simulink model "scattering_pos_pos_denis_2022a"  (R2022a)
settings: Solver=VariableStepAuto  StartTime=0.0  StopTime=10.0  RelTol=1e-3
values from neighbouring files (symbols this model uses):
  A = 2    [scattering_params.m]    (also in scattering_params_force_pos.m = 3; scattering_params_pos_pos.m = 3)
  b = 1    [scattering_params.m]    (also in scattering_params_force_pos.m = 40; scattering_params_pos_pos.m = 100)
  Be = 100    [scattering_params.m]    (also in scattering_params_force_pos.m; scattering_params_pos_pos.m)
  Bh = 1.5    [scattering_params.m]    (also in scattering_params_force_pos.m = 1; scattering_params_pos_pos.m = 1)
  Dh = 0.1    [scattering_params.m]    (also in scattering_params_force_pos.m = 16; scattering_params_pos_pos.m = 16)
  discrete_delay = 100    [scattering_params_force_pos.m]    (also in scattering_params_pos_pos.m)
  Dm = 0    [scattering_params.m]    (also in scattering_params_force_pos.m; scattering_params_pos_pos.m)
  Ds = 0    [scattering_params.m]    (also in scattering_params_force_pos.m; scattering_params_pos_pos.m)
  Fc = 1    [scattering_params.m]    (also in scattering_params_force_pos.m = 0.25; scattering_params_pos_pos.m = 0.25)
  Flp = 5    [scattering_params.m]    (also in scattering_params_force_pos.m = 0.5; scattering_params_pos_pos.m = 0.5)
  Jh = 1    [scattering_params.m]    (also in scattering_params_force_pos.m; scattering_params_pos_pos.m)
  Ke = 200    [scattering_params.m]    (also in scattering_params_force_pos.m; scattering_params_pos_pos.m)
  Mm = 0.5    [scattering_params.m]    (also in scattering_params_force_pos.m; scattering_params_pos_pos.m)
  Ms = 2    [scattering_params.m]    (also in scattering_params_force_pos.m; scattering_params_pos_pos.m)
  Ph = 10    [scattering_params.m]    (also in scattering_params_force_pos.m; scattering_params_pos_pos.m)
  scattering_filter_freq = 10    [scattering_params.m]    (also in scattering_params_force_pos.m; scattering_params_pos_pos.m)
  Ts = 0.001    [scattering_params_force_pos.m]    (also in scattering_params_pos_pos.m)
  xe = 5    [scattering_params.m]    (also in scattering_params_force_pos.m = 2; scattering_params_pos_pos.m = 2)
settings Model: Creator=Manu  LastModifiedBy=Manu
settings ModelReferenceCC: EnableRefExpFcnMdlSchedulingChecks=off
settings RTWCC: Description=Generic Real-Time Target

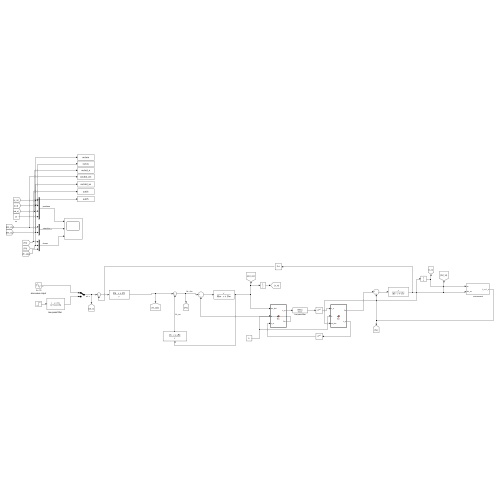
[thumbnail: Simulink's stored preview of the top-level diagram]
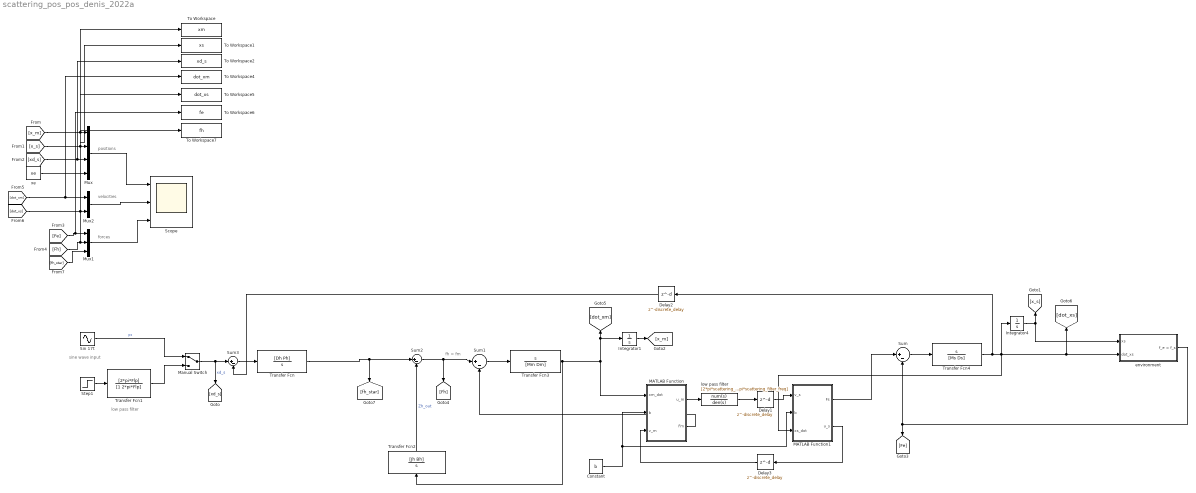
== system scattering_pos_pos_denis_2022a ==
  note: fh = fm
  note: sine wave input
  note: low pass filter
  note: positions
  note: forces
  note: velocities
  Constant : Constant  Value=b
  Delay1 : Delay  DelayLength=discrete_delay  SampleTime=Ts
  Delay2 : Delay  DelayLength=discrete_delay  SampleTime=Ts
  Delay3 : Delay  DelayLength=discrete_delay  SampleTime=Ts
  Integrator1 : Integrator
  Integrator4 : Integrator
  MATLAB Function : MATLAB Function  TreatAsAtomicUnit=on
  MATLAB Function1 : MATLAB Function  TreatAsAtomicUnit=on
  Manual Switch : ManualSwitch
  Mux : Mux
  Mux1 : Mux  Inputs=3
  Mux2 : Mux  Inputs=2
  Scope : Scope  NumInputPorts=3
  Sin 17t : Sin  Amplitude=A  Frequency=2*pi*Fc  SampleTime=0
  Step1 : Step  Time=0.5  After=A  SampleTime=0
  Sum{,1..3} (4 alike) : Sum  Inputs=|+-
  To Workspace : ToWorkspace  VariableName=xm  SaveFormat=Timeseries  SampleTime=-1
  To Workspace1 : ToWorkspace  VariableName=xs  SaveFormat=Timeseries  SampleTime=-1
  To Workspace2 : ToWorkspace  VariableName=xd_s  SaveFormat=Timeseries  SampleTime=-1
  To Workspace4 : ToWorkspace  VariableName=dot_xm  SaveFormat=Timeseries  SampleTime=-1
  To Workspace5 : ToWorkspace  VariableName=dot_xs  SaveFormat=Timeseries  SampleTime=-1
  To Workspace6 : ToWorkspace  VariableName=fe  SaveFormat=Timeseries  SampleTime=-1
  To Workspace7 : ToWorkspace  VariableName=fh  SaveFormat=Timeseries  SampleTime=-1
  Transfer Fcn : TransferFcn  Numerator=[Dh Ph]  Denominator=[1 0]
  Transfer Fcn1 : TransferFcn  Numerator=[2*pi*Flp]  Denominator=[1 2*pi*Flp]
  Transfer Fcn2 : TransferFcn  Numerator=[Jh Bh]  Denominator=[1 0]
  Transfer Fcn3 : TransferFcn  Numerator=[1 0]  Denominator=[Mm Dm]
  Transfer Fcn4 : TransferFcn  Numerator=[1 0]  Denominator=[Ms Ds]
  environment : Subsystem
  low pass filter : TransferFcn  Numerator=[2*pi*scattering_filter_freq]  Denominator=[1 2*pi*scattering_filter_freq]
  xe : Constant  Value=xe
  wires:
  Manual Switch/1 -> Sum3/1, [xd_s]  "xd_s"
  Transfer Fcn2/1 -> Sum2/2  "Zh_out"
  Sin 17t/1 -> Manual Switch/1  "F*"
  Transfer Fcn1/1 -> Manual Switch/2
  Step1/1 -> Transfer Fcn1/1
  Sum2/1 -> [Fh], Sum1/1
  Sum1/1 -> Transfer Fcn3/1
  Sum/1 -> Transfer Fcn4/1
  Transfer Fcn4/1 -> MATLAB Function1/3(xs_dot), [dot_xs], environment/2(dot_xs), Integrator4/1, Delay2/1
  environment/1(f_e = f_s) -> [Fe], Sum/2
  Transfer Fcn3/1 -> Transfer Fcn2/1, [dot_xm], Integrator1/1, MATLAB Function/1(xm_dot)
  [fh_star] -> Mux1/3
  Mux2/1 -> Scope/2
  [Fh] -> To Workspace7/1, Mux1/2
  [dot_xs] -> To Workspace5/1, Mux2/2
  [dot_xm] -> Mux2/1, To Workspace4/1
  [x_s] -> To Workspace1/1, Mux/2
  [x_m] -> To Workspace/1, Mux/1
  Mux1/1 -> Scope/3
  Mux/1 -> Scope/1
  xe/1 -> Mux/4
  [Fe] -> Mux1/1, To Workspace6/1
  [xd_s] -> To Workspace2/1, Mux/3
  Transfer Fcn/1 -> [fh_star], Sum2/1
  MATLAB Function/1(u_m) -> low pass filter/1
  Delay1/1 -> MATLAB Function1/1(v_s)
  MATLAB Function1/2(u_s) -> Delay3/1
  Delay3/1 -> MATLAB Function/3(v_m)
  MATLAB Function1/1(Fs) -> Sum/1
  MATLAB Function/2(Fm) -> Sum1/2
  Integrator4/1 -> environment/1(xs), [x_s]
  Sum3/1 -> Transfer Fcn/1
  Delay2/1 -> Sum3/2
  Integrator1/1 -> [x_m]
  Constant/1 -> MATLAB Function/2(b), MATLAB Function1/2(b)
  low pass filter/1 -> Delay1/1

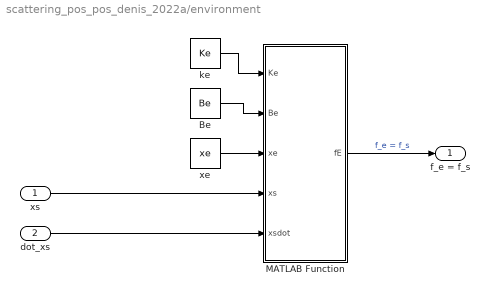
== system scattering_pos_pos_denis_2022a/environment ==
  xs : Inport
  dot_xs : Inport  Port=2
  Be : Constant  Value=Be
  MATLAB Function : MATLAB Function  TreatAsAtomicUnit=on
  ke : Constant  Value=Ke
  xe : Constant  Value=xe
  f_e = f_s : Outport
  wires:
  MATLAB Function/1(fE) -> f_e = f_s/1  "f_e = f_s"
  xs/1 -> MATLAB Function/4(xs)
  xe/1 -> MATLAB Function/3(xe)
  dot_xs/1 -> MATLAB Function/5(xsdot)
  ke/1 -> MATLAB Function/1(Ke)
  Be/1 -> MATLAB Function/2(Be)

== matlab function scattering_pos_pos_denis_2022a/MATLAB Function ==
  data: xm_dot input; b input; u_m output; v_m input; Fm output
function [u_m, Fm] = fcn(xm_dot, b, v_m)
u_m = sqrt(2*b)*xm_dot + v_m;
Fm = b*xm_dot + sqrt(2*b) * v_m;

== matlab function scattering_pos_pos_denis_2022a/environment/MATLAB Function ==
  data: Ke input; fE output; Be input; xe input; xs input; xsdot input
function fE = environment(Ke, Be, xe, xs, xsdot)
    if xs > xe
        fE = Ke * (xs - xe) + Be * xsdot; % Plot both contributions Ke and Be
    else
        fE = 0;
    end
end

== matlab function scattering_pos_pos_denis_2022a/MATLAB Function1 ==
  data: Fs output; v_s input; b input; xs_dot input; u_s output
function [Fs, u_s] = fcn(v_s, b, xs_dot)
u_s = -sqrt(2*b) * xs_dot + v_s;
Fs = -b*xs_dot + sqrt(2*b) * v_s;
